simulink model "Power_Electronics"  (Simulink 7.6)
settings: Solver=ode15s  StartTime=0.0  StopTime=10.0  FixedStep=0.01  MaxStep=0.2  RelTol=1e-3
libraries: fl_lib x27, nesl_utility x6, elec_lib x2, simulink x1
settings Model: Creator=Fodi  LastModifiedBy=Fodi

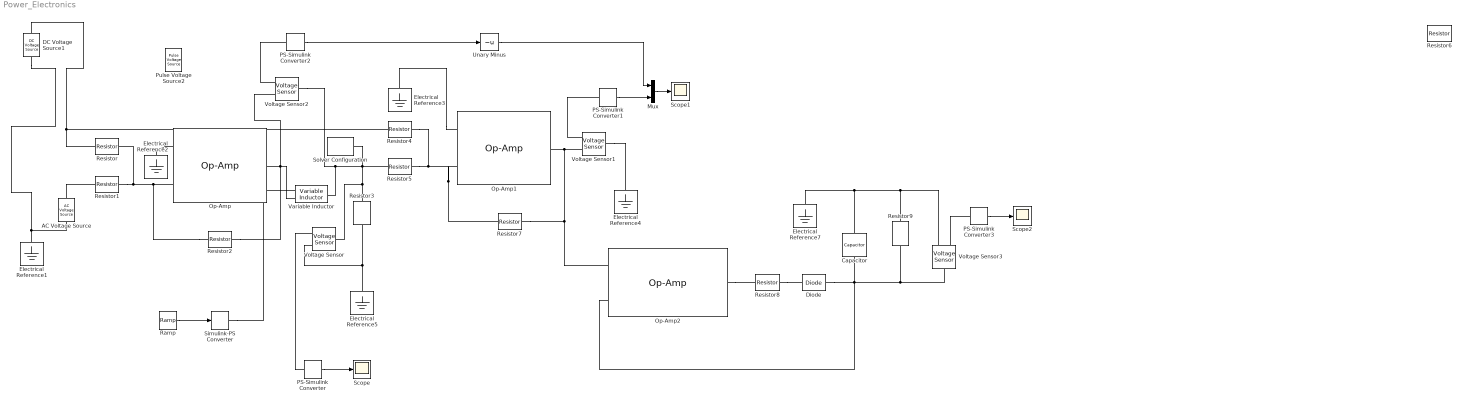
== system Power_Electronics ==
  AC Voltage Source : fl_lib/Electrical/Electrical Sources/AC Voltage Source  DialogController=NetworkEngine.DynNeDlgSource  SystemSampleTime=-1  amp=10 V  shift=0 rad  omega=500 Hz  i_Log=off  v_Log=off  LocalVarNames=|i|v  LocalVarDescs=|i|v  LocalVarLogging=[0 0]
  Capacitor : fl_lib/Electrical/Electrical Elements/Capacitor  DialogController=NetworkEngine.DynNeDlgSource  SystemSampleTime=-1  c=11 uF  v0=0 V  r=1e-6 Ohm  g=0 1/Ohm  i_Log=off  v_Log=off  vc_Log=off  LocalVarNames=|i|v|vc  LocalVarDescs=|i|v|Internal variable for voltage across capacitor term  LocalVarLogging=[0 0 0]
  DC Voltage Source1 : fl_lib/Electrical/Electrical Sources/DC Voltage Source  DialogController=NetworkEngine.DynNeDlgSource  SystemSampleTime=-1  v0=100 V  i_Log=off  v_Log=off  LocalVarNames=|i|v  LocalVarDescs=|i|v  LocalVarLogging=[0 0]
  Diode : fl_lib/Electrical/Electrical Elements/Diode  DialogController=NetworkEngine.DynNeDlgSource  SystemSampleTime=-1  Vf=0.6 V  Ron=0.3 Ohm  Goff=1e-8 1/Ohm  i_Log=off  v_Log=off  LocalVarNames=|i|v  LocalVarDescs=|i|v  LocalVarLogging=[0 0]
  Electrical Reference{1..5,7} (6 alike) : fl_lib/Electrical/Electrical Elements/Electrical Reference  DialogController=NetworkEngine.DynNeDlgSource  SystemSampleTime=-1  i_Log=off  LocalVarNames=|i  LocalVarDescs=|i  LocalVarLogging=0
  Mux : Mux  Inputs=2
  Op-Amp : fl_lib/Electrical/Electrical Elements/Op-Amp  DialogController=NetworkEngine.DynNeDlgSource  SystemSampleTime=-1  i1_Log=off  v1_Log=off  outI_Log=off  LocalVarNames=|i1|v1|outI  LocalVarDescs=|i1|v1|outI  LocalVarLogging=[0 0 0]
  Op-Amp1 : fl_lib/Electrical/Electrical Elements/Op-Amp  DialogController=NetworkEngine.DynNeDlgSource  SystemSampleTime=-1  i1_Log=off  v1_Log=off  outI_Log=off  LocalVarNames=|i1|v1|outI  LocalVarDescs=|i1|v1|outI  LocalVarLogging=[0 0 0]
  Op-Amp2 : fl_lib/Electrical/Electrical Elements/Op-Amp  DialogController=NetworkEngine.DynNeDlgSource  SystemSampleTime=-1  i1_Log=off  v1_Log=off  outI_Log=off  LocalVarNames=|i1|v1|outI  LocalVarDescs=|i1|v1|outI  LocalVarLogging=[0 0 0]
  PS-Simulink Converter{,1..3} (4 alike) : nesl_utility/PS-Simulink Converter  DialogController=NetworkEngine.DynNeUtilDlgSource  SystemSampleTime=-1  PhysicalDomain=network_engine_domain  LeftPortType=input  RightPortType=output  SubClassName=ps_output  Unit=1  AffineConversion=off
  Pulse Voltage Source2 : elec_lib/Additional Components/SPICE-Compatible Components/Sources/Pulse Voltage Source  DialogController=NetworkEngine.DynNeDlgSource  SystemSampleTime=-1  V1=0 V  V2=100 V  TD=0 s  TR=1e-9 s  TF=1e-9 s  PW=1.5 ms  PER=2 ms  voltage_Log=off  LocalVarNames=|voltage  LocalVarDescs=|Voltage (V)  LocalVarLogging=0
  Ramp : simulink/Sources/Ramp  SystemSampleTime=-1  slope=0.1  start=0  X0=0
  Resistor{,1..2,4..7} (7 alike) : fl_lib/Electrical/Electrical Elements/Resistor  DialogController=NetworkEngine.DynNeDlgSource  SystemSampleTime=-1  R=1 kOhm  i_Log=off  v_Log=off  LocalVarNames=|i|v  LocalVarDescs=|i|v  LocalVarLogging=[0 0]
  Resistor3 : fl_lib/Electrical/Electrical Elements/Resistor  DialogController=NetworkEngine.DynNeDlgSource  SystemSampleTime=-1  R=100 Ohm  i_Log=off  v_Log=off  LocalVarNames=|i|v  LocalVarDescs=|i|v  LocalVarLogging=[0 0]
  Resistor8 : fl_lib/Electrical/Electrical Elements/Resistor  DialogController=NetworkEngine.DynNeDlgSource  SystemSampleTime=-1  R=100 Ohm  i_Log=off  v_Log=off  LocalVarNames=|i|v  LocalVarDescs=|i|v  LocalVarLogging=[0 0]
  Resistor9 : fl_lib/Electrical/Electrical Elements/Resistor  DialogController=NetworkEngine.DynNeDlgSource  SystemSampleTime=-1  R=11 kOhm  i_Log=off  v_Log=off  LocalVarNames=|i|v  LocalVarDescs=|i|v  LocalVarLogging=[0 0]
  Scope : Scope
  Scope1 : Scope
  Scope2 : Scope
      settings: SaveName=ScopeData2
  Simulink-PS Converter : nesl_utility/Simulink-PS Converter  DialogController=NetworkEngine.DynNeUtilDlgSource  SystemSampleTime=-1  PhysicalDomain=network_engine_domain  LeftPortType=input  RightPortType=output  SubClassName=ps_input  Unit=1  AffineConversion=off  InputFilterTimeConstant=.001  UdotUserProvided=0
  Solver Configuration : nesl_utility/Solver Configuration  DialogController=NetworkEngine.DynNeUtilDlgSource  SystemSampleTime=-1  PhysicalDomain=network_engine_domain  LeftPortType=input  RightPortType=generic  SubClassName=solver  Accelerate=off  Profile=off  ResidualTolerance=1e-9  MaxNonlinIter=3  MaxModeIter=2  DoFixedCost=off  UseLocalSampling=off  DoDC=off  LinearAlgebra=Sparse  LocalSolverSampleTime=.001  LocalSolverChoice=NE_BACKWARD_EULER_ADVANCER  UseLocalSolver=off
  Unary Minus : UnaryMinus
  Variable Inductor : elec_lib/Passive Devices/Variable Inductor  DialogController=NetworkEngine.DynNeDlgSource  SystemSampleTime=-1  prm=1  Lmin=1e-6 H  g=1e-9 1/Ohm  i0=0 A  phi0=0 Wb  LocalVarLogging=[]
  Voltage Sensor{,1..3} (4 alike) : fl_lib/Electrical/Electrical Sensors/Voltage Sensor  DialogController=NetworkEngine.DynNeDlgSource  SystemSampleTime=-1  i1_Log=off  v1_Log=off  LocalVarNames=|i1|v1  LocalVarDescs=|i1|v1  LocalVarLogging=[0 0]
  wires:
  PS-Simulink Converter/1 -> Scope/1
  PS-Simulink Converter1/1 -> Mux/2
  PS-Simulink Converter2/1 -> Unary Minus/1
  Mux/1 -> Scope1/1
  Unary Minus/1 -> Mux/1
  PS-Simulink Converter3/1 -> Scope2/1
  Ramp/1 -> Simulink-PS Converter/1
  connections:
  Resistor2/LConn1 -- Resistor/RConn1 -- Resistor1/RConn1 -- Op-Amp/LConn2
  Variable Inductor/LConn2 -- Op-Amp/RConn1 -- Resistor2/RConn1 -- Voltage Sensor2/RConn2
  Op-Amp/LConn1 -- Electrical Reference2/LConn1
  AC Voltage Source/LConn1 -- Resistor1/LConn1
  Resistor5/RConn1 -- Resistor7/LConn1 -- Op-Amp1/LConn2 -- Resistor4/RConn1
  Resistor7/RConn1 -- Op-Amp1/RConn1 -- Voltage Sensor1/RConn2 -- Op-Amp2/LConn1
  Voltage Sensor1/LConn1 -- Electrical Reference4/LConn1
  Voltage Sensor1/RConn1 -- PS-Simulink Converter1/LConn1
  Electrical Reference3/LConn1 -- Op-Amp1/LConn1
  Voltage Sensor2/LConn1 -- Resistor5/LConn1 -- Solver Configuration/RConn1 -- Resistor3/LConn1 -- Voltage Sensor/LConn1 -- Variable Inductor/RConn1
  Voltage Sensor/RConn1 -- PS-Simulink Converter/LConn1
  Voltage Sensor/RConn2 -- Resistor3/RConn1 -- Electrical Reference5/LConn1
  Voltage Sensor2/RConn1 -- PS-Simulink Converter2/LConn1
  DC Voltage Source1/LConn1 -- Resistor/LConn1 -- Resistor4/LConn1
  DC Voltage Source1/RConn1 -- Electrical Reference1/LConn1 -- AC Voltage Source/RConn1
  Resistor8/RConn1 -- Diode/LConn1
  Resistor9/RConn1 -- Diode/RConn1 -- Capacitor/LConn1 -- Op-Amp2/LConn2 -- Voltage Sensor3/LConn1
  Resistor9/LConn1 -- Voltage Sensor3/RConn2 -- Capacitor/RConn1 -- Electrical Reference7/LConn1
  Voltage Sensor3/RConn1 -- PS-Simulink Converter3/LConn1
  Simulink-PS Converter/RConn1 -- Variable Inductor/LConn1
  Op-Amp2/RConn1 -- Resistor8/LConn1
